simulink model "uz_ParameterID_6ph"  (R2021b)
settings: Solver=FixedStepDiscrete  StartTime=0.0  StopTime=160  FixedStep=0.000005  RelTol=1e-3  EnableMultiTasking=on
model workspace (MATLAB code in the model file):
  | cmdLim = Simulink.Parameter;
  | cmdLim.Value = 15;
  | cmdLim.Description = 'Limit for controlling the maximum surface command angle.';
  | cmdLim.Min = 0;
  | cmdLim.Max = 90;
  | cmdLim.DocUnits = 'deg';
  | 
  | dispGain = Simulink.Parameter;
  | dispGain.Value = 0.75;
  | dispGain.Description = 'Gain applied to the displacement error.';
  | dispGain.Min = 0;
  | dispGain.Max = [];
  | dispGain.DocUnits = 'deg/sec/deg';
  | 
  | dispLim = Simulink.Parameter;
  | dispLim.Value = 30;
  | dispLim.Description = 'Limit for controlling the maximum commanded angle.';
  | dispLim.Min = 0;
  | dispLim.Max = 180;
  | dispLim.DocUnits = 'deg';
  | 
  | intGain = Simulink.Parameter;
  | intGain.Value = 0.5;
  | intGain.Description = 'Gain applied to the integral error.';
  | intGain.Min = 0;
  | intGain.Max = [];
  | intGain.DocUnits = 'deg/sec/deg/sec';
  | 
  | intLim = Simulink.Parameter;
  | intLim.Value = 5;
  | intLim.Description = 'Limit for controlling the maximum commanded angle.';
  | intLim.Min = 0;
  | intLim.Max = 90;
  | intLim.DocUnits = 'deg';
  | 
  | rateGain = Simulink.Parameter;
  | rateGain.Value = 2;
  | rateGain.Description = 'Gain applied to the rate error.';
  | rateGain.Min = 0;
  | rateGain.Max = [];
  | rateGain.DocUnits = 'deg/deg/sec';
  | 
  | rateLim = Simulink.Parameter;
  | rateLim.Value = 6;
  | rateLim.Description = 'Limit for controlling the maximum commanded angle.';
  | rateLim.Min = 0;
  | rateLim.Max = 180;
  | rateLim.DocUnits = 'deg/sec';
  | 
  | hdgGain = Simulink.Parameter;
  | hdgGain.Value = 0.015;
values from neighbouring files (symbols this model uses):
  d_f_states = 20000    [Parameter_Init_Buehler_201.m]
  d_I_n = 8    [Parameter_Init_Buehler_201.m]
  d_Ki_id = 162.47    [Parameter_Init_Buehler_201.m]
  d_Ki_iq = 162.47    [Parameter_Init_Buehler_201.m]
  d_Ki_n = 1.982    [Parameter_Init_Buehler_201.m]
  d_Kp_id = 0.369    [Parameter_Init_Buehler_201.m]
  d_Kp_iq = 0.369    [Parameter_Init_Buehler_201.m]
  d_Kp_n = 0.198    [Parameter_Init_Buehler_201.m]
  d_L_d = 0.00031    [Parameter_Init_Buehler_201.m]
  d_L_q = 0.00033    [Parameter_Init_Buehler_201.m]
  d_n_n = 3200    [Parameter_Init_Buehler_201.m]
  d_p = 4    [Parameter_Init_Buehler_201.m]
  d_psi_pm = 0.0075    [Parameter_Init_Buehler_201.m]
  d_R_ph = d_R_ph_ph/2    (= 0.089)    [Parameter_Init_Buehler_201.m]
undefined symbols (not defined in the file or in its folder): i_dq_ref, n_ref
(part 1 of 2)
settings Model: RequirementInfo={} %GIDa_fe9045fd_0412_4b6e_8206_617cc20e6fde  FPTRunName=Active  Creator=ts  LastModifiedBy=valen
settings SolverCC: AlgebraicLoopSolver=TrustRegion  PositivePriorityOrder=on  AutoInsertRateTranBlk=on
settings DataIOCC: SaveOutput=off  SignalLogging=off  DSMLogging=off  SaveTime=off
settings OptimizationCC: DefaultParameterBehavior=Inlined  UseDivisionForNetSlopeComputation=on  GainParamInheritBuiltInType=on  UseFloatMulNetSlope=on  DefaultUnderspecifiedDataType=single  UseSpecifiedMinMax=on  InlineInvariantSignals=on  PassReuseOutputArgsAs=Individual arguments  ZeroExternalMemoryAtStartup=off  ZeroInternalMemoryAtStartup=off  NoFixptDivByZeroProtection=on  EfficientFloat2IntCast=on  LifeSpan=1  MaxStackSize=64  OptimizeBlockOrder=speed  DifferentSizesBufferReuse=on  EfficientTunableParamExpr=on
settings DebuggingCC: BusObjectLabelMismatch=error  AllowSymbolicDim=off  SFUnexpectedBacktrackingDiag=warning  SFNoUnconditionalDefaultTransitionDiag=warning  SFExecutionAtInitializationDiag=none  SFMachineParentedDataDiag=warning  ArithmeticOperatorsInVariantConditions=warning
settings HardwareCC: ProdBitPerPointer=32  ProdBitPerSizeT=32  ProdBitPerPtrDiffT=32  ProdLargestAtomicInteger=Long  ProdLargestAtomicFloat=Double  ProdWordSize=32  ProdLongLongMode=on  ProdHWDeviceType=ARM Compatible->ARM Cortex-R  HardwareBoardFeatureSet=SoCBlockset
settings SFSimCC: SimGenImportedTypeDefs=on  MATLABDynamicMemAlloc=off
settings RTWCC: Description=Embedded Coder  SystemTargetFile=ert.tlc  GenCodeOnly=on  TemplateMakefile=ert_default_tmf  GenerateReport=on  BuildConfiguration=Faster Runs  IncludeHyperlinkInReport=on  LaunchReport=on  GenerateTraceInfo=on  GenerateTraceReport=on  GenerateTraceReportSl=on  GenerateTraceReportSf=on  GenerateTraceReportEml=on  GenerateCodeMetricsReport=on  CheckMdlBeforeBuild=Warning
settings CodeAppCC: ForceParamTrailComments=on  IgnoreCustomStorageClasses=off  OperatorAnnotations=on  SimulinkDataObjDesc=on  SFDataObjDesc=on  MATLABFcnDesc=on  CustomSymbolStrGlobalVar=rt$M$R$N  CustomSymbolStrType=$N$M$R_t  CustomSymbolStrFcn=$N$M$F  CustomSymbolStrMacro=$N$M  InsertBlockDesc=on  StateflowObjectComments=on  MATLABSourceComments=on  EnableCustomComments=on  ReqsInCode=on
settings ERTTargetCC: TargetLangStandard=C99 (ISO)  CodeReplacementLibrary=GNU C99 extensions  MultiwordLength=2048  IncludeMdlTerminateFcn=off  CombineSignalStateStructs=on  SuppressErrorStatus=on  IncludeFileDelimiter=UseQuote  SupportAbsoluteTime=off  CodeInterfacePackaging=Reusable function  RemoveResetFunc=off  InlinedParameterPlacement=NonHierarchical  MultiInstanceErrorCode=Warning  RootIOFormat=Part of model data structure  ERTCustomFileTemplate=example_file_process.tlc  GlobalDataDefinition=InSourceFile  GlobalDataReference=InSourceFile  ERTFilePackagingFormat=CompactWithDataFile
settings ConfigComp: CovScope=ReferencedModels  CovSaveName=covdata_rollAP  CovMetricSettings=dcmtrwe  CovHTMLOptions=-sRT=1 -aTS=1 -bRG=1 -bTC=1 -hTR=1 -nFC=0 -scm=1 -bcm=1 -xEv=0  CovSaveCumulativeToWorkspaceVar=on  CovSaveSingleToWorkspaceVar=on  CovCumulativeVarName=covCumulativeData_rollAP  CovReportOnPause=off  CovExternalEMLEnable=off  CovSFcnEnable=off

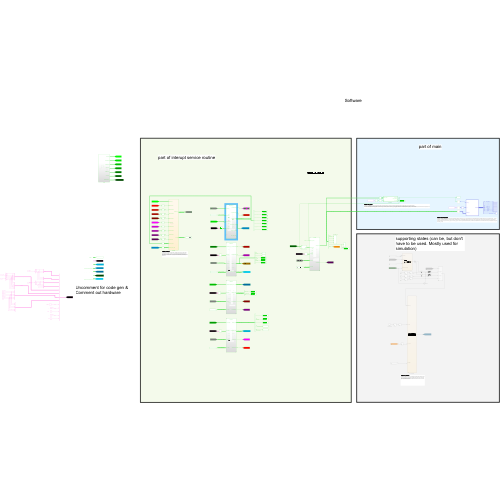
[thumbnail: Simulink's stored preview of the top-level diagram]
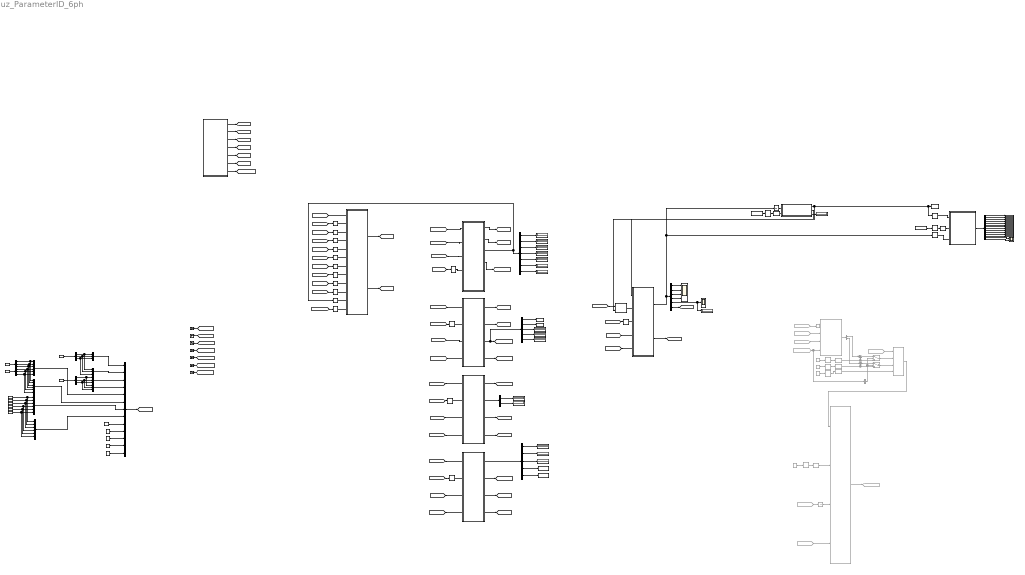
== system uz_ParameterID_6ph ==
  note: Description of Interpoaltion_Mesh_Grid:
      |
      | This function is calculating the regular flux maps out of the irregular scatter data array stored in psi_array_in. The outputs rangeX are containg the flux maps axis information, whereby the range is related to 3 times "i_rat" input.
      | Furthermore, the temperature dependency of the permanent flux is calculated if there are enough measuring values stored in the "delta_psi" array. The temperature constant as well as the estimated error of permanent flux,
      | at reference temperature, are given out on "psi_temp_const" and "psi_temp_error" outputs. Using this temperature dependency, the flux maps are updated with the permanent flux offset caused by the temperature which is given
      | in on "Wtemp_in" input.
  note: Stateflow for OnlineID
  note: part of main
  note: part of interupt service routine
  note: Software
  note: Description of clean_psi_array:
      |
      | This function is cleaning the array storing the measurement values, which always consits of a d-q-current combination a winding temperature and a speed value such as a d-q-flux combination
      | The function is searching for measuring pairs which are closer than "eta_c" to their neighbours. In this case it is averaging this similar pairs to avoid measuring values containing the same information.
      | This is essential for calculating a wide ranging flux map out of this array. Furthermore, there is an output "n_flux_points" giving back the amount of independent measuring pairs. This is the number (x/100) i show in the JavaGUI on the rigth top corner.
  note: Uncomment for code gen & Comment out hardware
  note: Description of ControlState:
      |
      | This state includes controls all the other states. It decides, based on user input, which state is executed and in which order. This is done via ControlFlags and finished/entered Flags of the individual states. If multiple ID's are requested, this state will automatically start the next one after the previous one has finished. This is an integral part of the ParameterID and must always be implemented.
  note: Description FOC_ControlState:
      |
      | This Stateflow is entered, after every other ID-state is finished (except OnlineID). It's just a simple state for current & speed control, depending on what the user chose in the config. This is only used to control the FOC with inputs after the ID-states are done. This state is solely used for simulation purposes.
  note: supporting states (can be, but don't have to be used. Mostly used for simulation)
  0 = current control 1 = speed control : Constant  Commented=on  Value=0
  AutoRefCurrents : Stateflow chart  Commented=on  TreatAsAtomicUnit=on
      settings: PortSchema="{\"entries\":[{\"content\":{\"sides\":[{\"content\":{\"connectorIds\":[\"In1\",\"In2\",\"In4\",\"In3\"]},\"type\":\"ConnectorPlacement.EquallySpacedRectSide\",\"uuid\":\"72ec0a24-315d-4dd0-9768-288ce3b452e0\"},{\"content\":{\"connectorIds\":[\"Out1\"],\"side\":\"RIGHT\"},\"type\":\"ConnectorPlacement.EquallySpacedRectSide\",\"uuid\":\"ab2b6233-d9cb-4afd-91e6-1fd664e04fd4\"},{\"content\":{\"connectorIds\":[],\"side\":\"TOP\"},\"type\":\"ConnectorPlacement.EquallySpacedRectSide\",\"uuid\":\"64b2df27-0928-499d-b44c-d4351b3511f9\"}]},\"type\":\"ConnectorPlacement.EquallySpacedConnector\",\"uuid\":\"4bb55e1f-14f7-4ef2-bb52-ee940a9b3e5d\"}],\"packageUris\":[\"http://schema.mathworks.com/mf0/Connector/R2020b\"],\"version\":\"1.0\"}"
  Bus Assignment : BusAssignment  Commented=on  AssignedSignals=i_dq_ref.d,i_dq_ref.q,n_ref
  Bus Assignment1 : BusAssignment  AssignedSignals=array_cleaned
  Bus Creator : BusCreator  Inputs=13  OutDataTypeStr=Bus: uz_ParaID_ActualValues_t
  Bus Creator1 : BusCreator  Inputs=3  OutDataTypeStr=Bus: uz_3ph_abc_t
  Bus Creator10 : BusCreator  Inputs=6  OutDataTypeStr=Bus: uz_6ph_abc_t
  Bus Creator11 : BusCreator  Inputs=6  OutDataTypeStr=Bus: uz_6ph_abc_t
  Bus Creator2 : BusCreator  Inputs=3  OutDataTypeStr=Bus: uz_3ph_abc_t
  Bus Creator3 : BusCreator  Inputs=6  OutDataTypeStr=Bus: uz_6ph_dq_t
  Bus Creator4 : BusCreator  Inputs=6  OutDataTypeStr=Bus: uz_6ph_dq_t
  Bus Creator5 : BusCreator  Inputs=3  OutDataTypeStr=Bus: uz_3ph_dq_t
  Bus Creator6 : BusCreator  Inputs=3  OutDataTypeStr=Bus: uz_3ph_dq_t
  Bus Selector : BusSelector  OutputSignals=BrkTorque,CoulTorque,ViscoTorque,measArrayTorque,measArraySpeed
  Bus Selector2 : BusSelector  OutputSignals=thetaOffset,PMSM_parameters.R_ph_Ohm,PMSM_parameters.Ld_Henry,PMSM_parameters.Lq_Henry,PMSM_parameters.Psi_PM_Vs,PMSM_parameters.J_kg_m_squared,PMSM_parameters.polePairs
  Bus Selector3 : BusSelector  OutputSignals=range_psid_X,range_psiq_X,range_id_X,range_iq_X,range_psid_Y,range_psiq_Y,range_id_Y,range_iq_Y,psiq_grid,psid_grid,id_grid,iq_grid,psi_temp_const,psi_temp_error
  Bus Selector4 : BusSelector  Commented=on  OutputSignals=i_dq_ref.d,i_dq_ref.q
  Bus Selector5 : BusSelector  OutputSignals=R_s,WindingTemp
  Bus Selector6 : BusSelector  OutputSignals=c_est_out,d_est_out,LoadInertia,TrainInertia,rotorInertia
  Bus Selector7 : BusSelector  Commented=on  OutputSignals=enableCRS
  Bus Selector8 : BusSelector  OutputSignals=Rph_out,Ld_out,Lq_out,psi_pm_out,activeState,id_out
  CleanPsiArray : MATLAB Function
  Const27 : Constant  Value=0.01*d_I_n
  Const53 : Constant  Value=d_I_n
  Const7 : Constant  Commented=on  Value=0.6
  Const8 : Constant  Commented=on  Value=0
  Const9 : Constant  Commented=on  Value=1000
  Constant{,2..5,7} (6 alike) : Constant  Value=0  OutDataTypeStr=single
  Constant{1,6,16..17} (4 alike) : Constant  Value=[0;0;0]  OutDataTypeStr=single
  ControlState : Stateflow chart  TreatAsAtomicUnit=on
      settings: PortSchema="{\"entries\":[{\"content\":{\"sides\":[{\"content\":{\"connectorIds\":[\"In11\",\"In1\",\"In2\",\"In3\",\"In4\",\"In5\",\"In8\",\"In7\",\"In6\",\"In12\",\"In9\",\"In10\"]},\"type\":\"ConnectorPlacement.EquallySpacedRectSide\",\"uuid\":\"3338e9a8-28b4-45bb-be16-581ebbf0e7d5\"},{\"content\":{\"connectorIds\":[\"Out1\",\"Out2\"],\"side\":\"RIGHT\"},\"type\":\"ConnectorPlacement.EquallySpacedRectSide\",\"uuid\":\"68ffdf0a-d88e-422d-a36e-256c991e1a1a\"},{\"content\":{\"connectorIds\":[],\"side\":\"TOP\"},\"type\":\"ConnectorPlacement.EquallySpacedRectSide\",\"uuid\":\"571bf6fb-233c-470d-b735-d23e4cf83e69\"}]},\"type\":\"ConnectorPlacement.EquallySpacedConnector\",\"uuid\":\"829c5db0-50d3-4caf-9d4e-ee907b3905d4\"}],\"packageUris\":[\"http://schema.mathworks.com/mf0/Connector/R2020b\"],\"version\":\"1.0\"}"
  Data Type Conversion107 : DataTypeConversion  Commented=on  OutDataTypeStr=boolean
  Data Type Conversion12 : DataTypeConversion  Commented=on  OutDataTypeStr=single
  Data Type Conversion13 : DataTypeConversion  Commented=on  OutDataTypeStr=single
  Data Type Conversion15 : DataTypeConversion  Commented=on  OutDataTypeStr=single
  Data Type Conversion60 : DataTypeConversion  OutDataTypeStr=single
  Data Type Conversion86 : DataTypeConversion  OutDataTypeStr=single
  Delay{,1..9,14} (11 alike) : Delay  DelayLength=1  InitialCondition=0
  Demux{1..4} (4 alike) : Demux  Outputs=3
  Display{1..3,5..11} (10 alike) : Display
  ElectricalID6ph : Subsystem  ReferencedSubsystem=ElectricalID_6ph
  FOC_ControlState : Stateflow chart  Commented=on  TreatAsAtomicUnit=on
      settings: PortSchema="{\"entries\":[{\"content\":{\"sides\":[{\"content\":{\"connectorIds\":[\"In2\",\"In4\",\"In1\",\"In3\"]},\"type\":\"ConnectorPlacement.EquallySpacedRectSide\",\"uuid\":\"51616e24-a97c-4867-a832-fbf8995ba5af\"},{\"content\":{\"connectorIds\":[\"Out1\"],\"side\":\"RIGHT\"},\"type\":\"ConnectorPlacement.EquallySpacedRectSide\",\"uuid\":\"f89ef2d6-1fe7-4143-9573-492fc01180c7\"},{\"content\":{\"connectorIds\":[],\"side\":\"TOP\"},\"type\":\"ConnectorPlacement.EquallySpacedRectSide\",\"uuid\":\"2a1663ee-9e4b-4188-8f87-b811d0bf4173\"}]},\"type\":\"ConnectorPlacement.EquallySpacedConnector\",\"uuid\":\"7415555a-a8a9-4dd7-91ae-86382220971a\"}],\"packageUris\":[\"http://schema.mathworks.com/mf0/Connector/R2020b\"],\"version\":\"1.0\"}"
  From11 : From  Commented=on  GotoTag=OnlineID_id_out
  From39 : From  Commented=on  GotoTag=ActualValues
  From40 : From  Commented=on  GotoTag=GlobalConfig
  From5 : From  Commented=on  GotoTag=ControlFlags
  From50 : From  Commented=on  GotoTag=GlobalConfig
  From51 : From  Commented=on  GotoTag=AutoRefCurrentsConfig
  From52 : From  Commented=on  GotoTag=ControlFlags
  Goto8 : Goto  Commented=on  GotoTag=FOCControl_output
  InterpMeshGrid : MATLAB Function  TreatAsAtomicUnit=on
  OnlineActiveState : Scope
  RT : RateTransition  Commented=on  OutPortSampleTime=0.0001
  Rate Transition : RateTransition  OutPortSampleTime=0.1
  Rate Transition{1,13..14,147} (4 alike) : RateTransition  Commented=on  OutPortSampleTime=1/d_f_states
  Rate Transition{2..6,78} (6 alike) : RateTransition  OutPortSampleTime=1/d_f_states
  Rate Transition85 : RateTransition  OutPortSampleTime=0.1
  Rate Transition90 : RateTransition  OutPortSampleTime=0.1
  Rs,Ld,Lq,Psi_pm : Scope  NumInputPorts=4
  Scope2 : Scope  NumInputPorts=2
  Subsystem Reference : Subsystem  ReferencedSubsystem=FrictionID
  Subsystem Reference1 : Subsystem  ReferencedSubsystem=FluxMapID
  Subsystem Reference3 : Subsystem  ReferencedSubsystem=TwoMassID
  Subsystem Reference4 : Subsystem  ReferencedSubsystem=OnlineID
  Sum : Sum  Commented=on  Inputs=|++
  Sum1 : Sum  Commented=on  Inputs=|++
  Switch2 : Switch  Commented=on  Criteria=u2 > Threshold
  Switch3 : Switch  Commented=on  Criteria=u2 > Threshold
  Terminator{,1..6} (7 alike) : Terminator
  To Workspace1 : ToWorkspace  VariableName=measArrayTorque  SampleTime=-1
      settings: MaxDataPoints=1
  To Workspace15 : ToWorkspace  VariableName=psi_array  SampleTime=-1
      settings: MaxDataPoints=1
  To Workspace16 : ToWorkspace  VariableName=rangepdX  SampleTime=-1
      settings: MaxDataPoints=1
  To Workspace17 : ToWorkspace  VariableName=rangepqX  SampleTime=-1
      settings: MaxDataPoints=1
  To Workspace18 : ToWorkspace  VariableName=rangeidX  SampleTime=-1
      settings: MaxDataPoints=1
  To Workspace19 : ToWorkspace  VariableName=rangeiqX  SampleTime=-1
      settings: MaxDataPoints=1
  To Workspace2 : ToWorkspace  VariableName=measArraySpeed  SampleTime=-1
      settings: MaxDataPoints=1
  To Workspace20 : ToWorkspace  VariableName=rangepdY  SampleTime=-1
      settings: MaxDataPoints=1
  To Workspace21 : ToWorkspace  VariableName=rangepqY  SampleTime=-1
      settings: MaxDataPoints=1
  To Workspace22 : ToWorkspace  VariableName=rangeidY  SampleTime=-1
      settings: MaxDataPoints=1
  To Workspace23 : ToWorkspace  VariableName=rangeiqY  SampleTime=-1
      settings: MaxDataPoints=1
  To Workspace24 : ToWorkspace  VariableName=psiq_grid  SampleTime=-1
      settings: MaxDataPoints=1
  To Workspace25 : ToWorkspace  VariableName=psid_grid  SampleTime=-1
      settings: MaxDataPoints=1
  To Workspace26 : ToWorkspace  VariableName=id_grid  SampleTime=-1
      settings: MaxDataPoints=1
  To Workspace27 : ToWorkspace  VariableName=iq_grid  SampleTime=-1
      settings: MaxDataPoints=1
  To Workspace31 : ToWorkspace  VariableName=c_est_out  SampleTime=-1
      settings: MaxDataPoints=1
  To Workspace32 : ToWorkspace  VariableName=d_est_out  SampleTime=-1
      settings: MaxDataPoints=1
  Unit Delay : UnitDelay  Commented=on  SampleTime=-1  HasFrameUpgradeWarning=on
  Unit Delay3 : UnitDelay  SampleTime=-1  HasFrameUpgradeWarning=on
  V_DC : Constant  Value=0  OutDataTypeStr=single
  config : Subsystem
  d-axis inductance Ld [H] : Display
  omega_el : Constant  Value=0  OutDataTypeStr=single
  omega_m : Constant  Value=0  OutDataTypeStr=single
  p : Display
  phase resistance [Ohm] : Display
  psiPM [Vs] : Display
  q-axis inductance Lq [H] : Display
  rotorInertia  [kg*m²] : Display
  thetaOffset [rad] : Display
  theta_el : Constant  Value=0  OutDataTypeStr=single
  theta_m : Constant  Value=0  OutDataTypeStr=single
  wires:
  Bus Selector/3 -> Display10/1  "<ViscoTorque>"
  Sum/1 -> Switch3/1
  Const8/1 -> Rate Transition13/1
  config/5(TwoMassIDConfig) -> [TwoMassIDConfig]
  Bus Selector2/4 -> q-axis inductance Lq [H]/1  "<Lq_Henry>"
  From40/1 -> AutoRefCurrents/2(GlobalConfig)
  [finishedFrictionID] -> Delay/1
  Delay/1 -> ControlState/1(finishedFrictionID)
  Bus Selector2/5 -> psiPM [Vs]/1  "<Psi_PM_Vs>"
  Bus Selector8/1 -> Rs,Ld,Lq,Psi_pm/1  "<Rph_out>"
  Bus Selector6/5 -> Display6/1  "<rotorInertia>"
  Sum1/1 -> Switch2/1
  Const9/1 -> Rate Transition1/1
  Rate Transition14/1 -> Data Type Conversion13/1
  config/1(GlobalConfig) -> [GlobalConfig_in]
  Delay14/1 -> ControlState/9(ElectricalID_output)
  Delay2/1 -> ControlState/6(enteredFluxMapID)
  Delay5/1 -> ControlState/8(enteredElectricalID)
  Delay6/1 -> ControlState/7(enteredTwoMassID)
  [enteredElectricalID] -> Delay5/1
  Rate Transition85/1 -> Data Type Conversion86/1
  [enteredFrictionID] -> Delay1/1
  Data Type Conversion13/1 -> Sum1/2, Switch2/3  "i_q_ref"
  Rate Transition90/1 -> InterpMeshGrid/3(OnlineID_input)
  [finishedFluxMapID] -> Delay4/1
  [finishedTwoMassID] -> Delay3/1
  From39/1 -> RT/1
  config/2(ElectricalIDConfig) -> [ElectricalIDConfig]
  config/4(FrictionIDConfig) -> [FrictionIDConfig]
  Const53/1 -> Rate Transition85/1
  Const27/1 -> Rate Transition78/1
  Data Type Conversion60/1 -> CleanPsiArray/2(eta_c)
  Bus Selector2/6 -> rotorInertia  [kg*m²]/1  "<J_kg_m_squared>"
  Bus Selector/1 -> Display11/1  "<BrkTorque>"
  Delay1/1 -> ControlState/5(enteredFrictionID)
  Bus Selector2/7 -> p/1  "<polePairs>"
  [ElectricalID_FOC_output] -> Delay8/1
  Rate Transition13/1 -> Data Type Conversion12/1
  Unit Delay/1 -> FOC_ControlState/1(i_d_Online_ref)
  Rate Transition/1 -> InterpMeshGrid/1(psi_array_in)
  Delay7/1 -> ControlState/2(finishedElectricalID)
  Bus Selector2/2 -> phase resistance [Ohm]/1  "<R_ph_Ohm>"
  Bus Selector2/3 -> d-axis inductance Ld [H]/1  "<Ld_Henry>"
  [ActualValues] -> Rate Transition6/1
  Delay8/1 -> ControlState/10(ElectricalID_FOC_output)
  Bus Selector6/3 -> Display3/1  "<LoadInertia>"
  ControlState/1(GlobalConfig_out) -> [GlobalConfig]
  [ActualValues] -> Rate Transition2/1
  config/6(OnlineIDConfig) -> [OnlineIDConfig]
  [ActualValues] -> Rate Transition3/1
  CleanPsiArray/2(array_cleaned_flag) -> Bus Assignment1/2
  Bus Selector5/1 -> Display1/1  "<R_s>"
  [GlobalConfig_in] -> ControlState/11(GlobalConfig_in)
  From5/1 -> FOC_ControlState/3(ControlFlags)
  Const7/1 -> Rate Transition14/1
  Bus Selector6/4 -> Display5/1  "<TrainInertia>"
  Data Type Conversion86/1 -> InterpMeshGrid/2(i_rat)
  Bus Selector8/4 -> Rs,Ld,Lq,Psi_pm/4  "<psi_pm_out>"
  Bus Selector8/2 -> Rs,Ld,Lq,Psi_pm/2  "<Ld_out>"
  Unit Delay3/1 -> CleanPsiArray/1(OnlineID_output)
  [OnlineIDConfig] -> Bus Assignment1/1
  Rate Transition78/1 -> Data Type Conversion60/1
  Rate Transition1/1 -> Data Type Conversion15/1
  Bus Selector8/5 -> Display8/1, OnlineActiveState/1  "<activeState>"
  Delay3/1 -> ControlState/3(finishedTwoMassID)
  CleanPsiArray/1(psi_array_out) -> Subsystem Reference4/1, Rate Transition/1, To Workspace15/1  "cleaned_psi_array"
  Bus Selector2/1 -> thetaOffset [rad]/1  "<thetaOffset>"
  config/3(FluxMapIDConfig) -> [FluxMapIDConfig]
  CleanPsiArray/3(n_flux_points) -> Display7/1
  Bus Selector/2 -> Display9/1  "<CoulTorque>"
  ControlState/2(ControlFlags) -> [ControlFlags]
  [ActualValues] -> Rate Transition4/1
  Bus Selector6/1 -> To Workspace31/1  "<c_est_out>"
  Bus Selector6/2 -> To Workspace32/1  "<d_est_out>"
  FOC_ControlState/1(FOCControl_output) -> Goto8/1
  Delay4/1 -> ControlState/4(finishedFluxMapID)
  [finishedElectricalID] -> Delay7/1
  Bus Assignment/1 -> FOC_ControlState/2(GlobalConfig)
  [ActualValues] -> Rate Transition5/1
  Bus Selector8/3 -> Rs,Ld,Lq,Psi_pm/3  "<Lq_out>"
  Data Type Conversion12/1 -> Switch3/3, Sum/2  "i_d_ref"
  [enteredFluxMapID] -> Delay2/1
  [enteredTwoMassID] -> Delay6/1
  Bus Selector5/2 -> Display2/1  "<WindingTemp>"
  [ActualValues] -> Terminator/1
  [TwoMassID_FOC_output] -> Terminator6/1
  [FrictionID_FOC_output] -> Terminator2/1
  [ElectricalID_FOC_output] -> Terminator3/1
  [FluxMapID_FOC_output] -> Terminator4/1
  [ControlFlags] -> Terminator1/1
  omega_el/1 -> Bus Creator/10  "omega_el"
  Bus Creator/1 -> [ActualValues]
  omega_m/1 -> Bus Creator/9  "omega_m"
  theta_m/1 -> Bus Creator/11  "theta_m"
  V_DC/1 -> Bus Creator/13  "V_DC"
  theta_el/1 -> Bus Creator/12  "theta_el"
  From50/1 -> Bus Assignment/1
  Switch2/1 -> Bus Assignment/3
  Switch3/1 -> Bus Assignment/2
  Data Type Conversion15/1 -> Bus Assignment/4  "n_ref"
  RT/1 -> AutoRefCurrents/1(ActualValues)
  Bus Selector8/6 -> [OnlineID_id_out]  "<id_out>"
  From11/1 -> Unit Delay/1
  Rate Transition147/1 -> Data Type Conversion107/1
  Data Type Conversion107/1 -> FOC_ControlState/4(controlType)  "controlType"
  0 = current control 1 = speed control/1 -> Rate Transition147/1
  Bus Selector3/1 -> To Workspace16/1  "<range_psid_X>"
  Bus Selector3/2 -> To Workspace17/1  "<range_psiq_X>"
  InterpMeshGrid/1(FluxMapData) -> Bus Selector3/1
  Bus Selector3/14 -> Scope2/2  "<psi_temp_error>"
  Bus Selector3/13 -> Scope2/1  "<psi_temp_const>"
  Bus Selector3/3 -> To Workspace18/1  "<range_id_X>"
  Bus Selector3/4 -> To Workspace19/1  "<range_iq_X>"
  Bus Selector3/5 -> To Workspace20/1  "<range_psid_Y>"
  Bus Selector3/6 -> To Workspace21/1  "<range_psiq_Y>"
  Bus Selector3/7 -> To Workspace22/1  "<range_id_Y>"
  Bus Selector3/8 -> To Workspace23/1  "<range_iq_Y>"
  Bus Selector3/9 -> To Workspace24/1  "<psiq_grid>"
  Bus Selector3/10 -> To Workspace25/1  "<psid_grid>"
  Bus Selector3/11 -> To Workspace26/1  "<id_grid>"
  Bus Selector3/12 -> To Workspace27/1  "<iq_grid>"
  config/7(AutoRefCurrentsconfig) -> [AutoRefCurrentsConfig]
  From51/1 -> Bus Selector7/1, AutoRefCurrents/3(AutoRefCurrentsConfig)
  AutoRefCurrents/1(AutoRefCurrents_output) -> Bus Selector4/1
  Bus Selector4/1 -> Sum/1  "<d>"
  Bus Selector4/2 -> Sum1/1  "<q>"
  Bus Selector7/1 -> Switch2/2, Switch3/2  "<enableCRS>"
  From52/1 -> AutoRefCurrents/4(ControlFlags)
  Delay9/1 -> ControlState/12(enteredOnlineID)
  [enteredOnlineID] -> Delay9/1
  Bus Selector/4 -> To Workspace1/1  "<measArrayTorque>"
  Bus Selector/5 -> To Workspace2/1  "<measArraySpeed>"
  [FrictionIDConfig] -> Subsystem Reference/1
  [GlobalConfig] -> Subsystem Reference/3
  [ControlFlags] -> Subsystem Reference/4
  Subsystem Reference/1 -> Bus Selector/1
  Subsystem Reference/2 -> [FrictionID_FOC_output]
  Subsystem Reference/3 -> [enteredFrictionID]
  Subsystem Reference/4 -> [finishedFrictionID]
  [FluxMapIDConfig] -> Subsystem Reference1/1
  [GlobalConfig] -> Subsystem Reference1/3
  [ControlFlags] -> Subsystem Reference1/4
  Subsystem Reference1/1 -> [FluxMapID_FOC_output]
  Subsystem Reference1/2 -> Bus Selector5/1
  Subsystem Reference1/3 -> [finishedFluxMapID]
  Subsystem Reference1/4 -> [enteredFluxMapID]
  ElectricalID6ph/3 -> Bus Selector2/1, Delay14/1
  [GlobalConfig] -> ElectricalID6ph/1
  [ControlFlags] -> ElectricalID6ph/2
  [ElectricalIDConfig] -> ElectricalID6ph/3
  Rate Transition6/1 -> ElectricalID6ph/4
  ElectricalID6ph/1 -> [enteredElectricalID]
  ElectricalID6ph/2 -> [finishedElectricalID]
  ElectricalID6ph/4 -> [ElectricalID_FOC_output]
  Subsystem Reference3/3 -> Bus Selector6/1, [TwoMassID_output]
  [TwoMassIDConfig] -> Subsystem Reference3/1
  [GlobalConfig] -> Subsystem Reference3/3
  [ControlFlags] -> Subsystem Reference3/4
  Subsystem Reference3/1 -> [finishedTwoMassID]
  Subsystem Reference3/2 -> [enteredTwoMassID]
  Subsystem Reference3/4 -> [TwoMassID_FOC_output]
  Subsystem Reference4/1 -> Unit Delay3/1, Rate Transition90/1, Bus Selector8/1
  Bus Assignment1/1 -> Subsystem Reference4/2
  Rate Transition3/1 -> Subsystem Reference4/3
  [GlobalConfig] -> Subsystem Reference4/4
  [ControlFlags] -> Subsystem Reference4/5
  Subsystem Reference4/2 -> [enteredOnlineID]
  Rate Transition2/1 -> Subsystem Reference3/2
  Rate Transition4/1 -> Subsystem Reference1/2
  Rate Transition5/1 -> Subsystem Reference/2
  Demux1/3 -> Bus Creator11/3, Bus Creator10/3  "c1"
  Demux1/2 -> Bus Creator11/2, Bus Creator10/2  "b1"
  Constant17/1 -> Demux2/1
  Constant16/1 -> Demux1/1
  Demux2/1 -> Bus Creator11/4, Bus Creator10/4  "a2"
  Demux2/3 -> Bus Creator11/6, Bus Creator10/6  "c2"
  Demux1/1 -> Bus Creator11/1, Bus Creator10/1  "a1"
  Demux2/2 -> Bus Creator11/5, Bus Creator10/5  "b2"
  Bus Creator11/1 -> Bus Creator/6  "i_abc_6ph"
  Bus Creator10/1 -> Bus Creator/5  "v_abc_6ph"
  Constant2/1 -> Bus Creator3/2, Bus Creator4/2  "q"
  Constant3/1 -> Bus Creator3/3, Bus Creator4/3  "x"
  Constant/1 -> Bus Creator3/1, Bus Creator4/1  "d"
  Bus Creator4/1 -> Bus Creator/7  "i_dq_6ph"
  Constant4/1 -> Bus Creator3/4, Bus Creator4/4  "y"
  Bus Creator3/1 -> Bus Creator/8  "v_dq_6ph"
  Constant5/1 -> Bus Creator3/5, Bus Creator4/5  "z1"
  Constant7/1 -> Bus Creator3/6, Bus Creator4/6  "z2"
  Demux3/3 -> Bus Creator2/3, Bus Creator1/3  "c"
  Demux3/1 -> Bus Creator2/1, Bus Creator1/1  "a"
  Demux3/2 -> Bus Creator2/2, Bus Creator1/2  "b"
  Constant1/1 -> Demux3/1
  Bus Creator1/1 -> Bus Creator/1  "V_abc"
  Bus Creator2/1 -> Bus Creator/2  "I_abc"
  Bus Creator5/1 -> Bus Creator/3  "i_dq"
  Constant6/1 -> Demux4/1
  Demux4/3 -> Bus Creator6/3, Bus Creator5/3  "zero"
  Demux4/1 -> Bus Creator6/1, Bus Creator5/1  "d"
  Demux4/2 -> Bus Creator6/2, Bus Creator5/2  "q"
  Bus Creator6/1 -> Bus Creator/4  "v_dq"
  [AutoRefCurrentsConfig] -> Terminator5/1

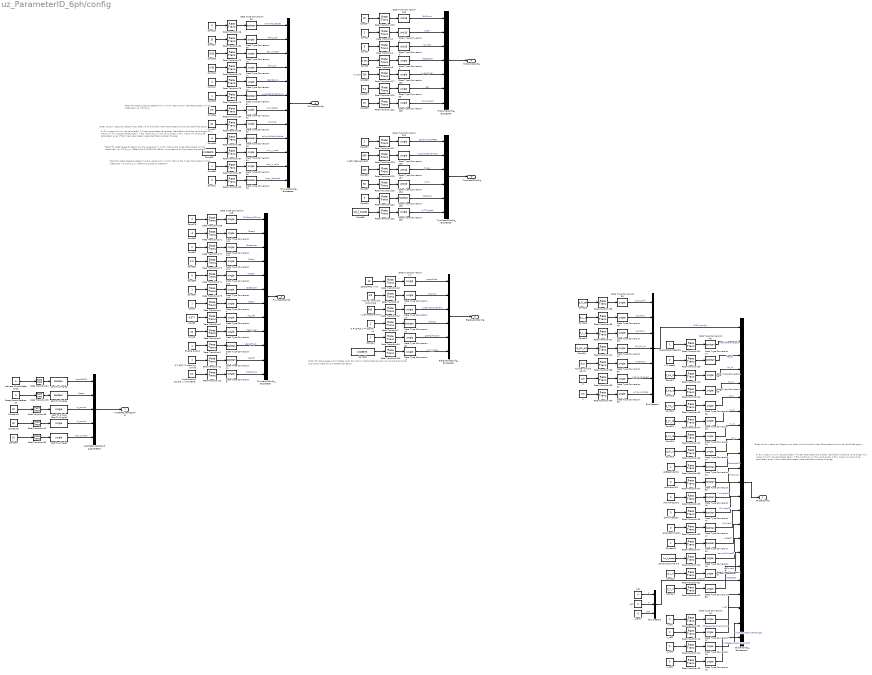
== system uz_ParameterID_6ph/config ==
  note: %1000
  note: Factor for rated speed,to determine the upper end in which interval the linear Parameters will
      | be measured. i.e. 0,5*d_n_n.
      | Default ist 0.625 for 2000rpm
  note: 0: Flux maps will only be calculated, if linear parameters have been identified inside the valid range.
      |     Flux maps will only be calculated again, if the machine is in the valid range.
      | 1:Flux maps will always be calculated, even if the linear parameters were identified outside of range.
  note: Enter value in seconds. Determines, after which time the linear Parameters have to be identified again.
  note: Factor for rated current,to determine in which interval the linear Parameters will
      | be measured. i.e. 0,5*d_I_n
  note: Factor for rated speed,to determine the lower end in which interval the linear Parameters will
      | be measured. i.e. 0,5*d_n_n.
      | Default ist 0.026875 for 86rpm (one rotation during measuring period)
  note: Factor for rated speed,which states when the rotor is rotating fast enough during the DutyCycle evaluation
      | Default ist 0.026875 for 86rpm
  note: 0: Flux maps will only be calculated, if linear parameters have been identified inside the valid range.
      |     Flux maps will only be calculated again, if the machine is in the valid range.
      | 1:Flux maps will always be calculated, even if the linear parameters were identified outside of range.
  note: Enter value in seconds. Determines, after which time the linear Parameters have to be identified again.
  "0 = Lq=Ld 1 = identify Lq " : Constant
  0 = off 1 = ident R_s online : Constant
  1 = reset1 : Constant  Value=0
  2 : Constant  Value=0.0
  3 : Constant  Value=0.0
  Activate ControlReference : Constant  Value=0  OutDataTypeStr=boolean
  Amplitude for SquareWave signal in d-current2 : Constant  Value=0.2
  AutoRefCurrentsConfig_Buscreator : BusCreator  Inputs=5  OutDataTypeStr=Bus: uz_ParaID_AutoRefCurrentsConfig_t
  Bus Creator1 : BusCreator  Inputs=7  OutDataTypeStr=Bus: uz_PMSM_t
  Bus Creator2 : BusCreator  Inputs=3  OutDataTypeStr=Bus: uz_3ph_dq_t
  Cast To Single : DataTypeConversion  OutDataTypeStr=single
  Cast To Single1 : DataTypeConversion  OutDataTypeStr=single
  Cast To Single2 : DataTypeConversion  OutDataTypeStr=single
  Cast To Single3 : DataTypeConversion  OutDataTypeStr=boolean
  Cast To Single4 : DataTypeConversion  OutDataTypeStr=boolean
  Const{1,47,78,81,91} (5 alike) : Constant  Value=2
  Const{10..11,58,83,94} (5 alike) : Constant  Value=0
  Const12 : Constant  Value=d_psi_pm
  Const13 : Constant  Value=d_I_n
  Const14 : Constant  Value=d_n_n
  Const16 : Constant  Value=d_L_d
  Const17 : Constant  Value=d_Kp_id
  Const18 : Constant  Value=d_Kp_iq
  Const19 : Constant  Value=d_Ki_iq
  Const2 : Constant  Value=5
  Const{4,20,28,60,84} (5 alike) : Constant
  Const21 : Constant  Value=d_Ki_id
  Const22 : Constant  Value=d_Kp_n
  Const23 : Constant  Value=d_Ki_n
  Const24 : Constant  Value=d_L_q
  Const25 : Constant  Value=d_R_ph
  Const3 : Constant  Value=0.001
  Const37 : Constant  Value=20
  Const43 : Constant  Value=0.05
  Const44 : Constant  Value=0.05
  Const5 : Constant  Value=0.077
  Const56 : Constant  Value=0.5
  Const57 : Constant  Value=20
  Const59 : Constant  Value=0.026875
  Const6 : Constant  Value=22
  Const62 : Constant  Value=0.026875
  Const64 : Constant  Value=0.2
  Const65 : Constant  Value=200
  Const67 : Constant  Value=20
  Const69 : Constant  Value=15
  Const80 : Constant  Value=-2
  Const82 : Constant  Value=0.0
  Const92 : Constant  Value=50
  Const93 : Constant  Value=400
  Const95 : Constant  Value=1/d_f_states
  Constant : Constant  Value=10
  Constant1 : Constant
  Constant3 : Constant  Value=20
  Constant4 : Constant  Value=20
  Data Type Conversion{1..2,103,136..137} (5 alike) : DataTypeConversion  OutDataTypeStr=uint16
  Data Type Conversion{8,10..11,23..24,26,40..41,43,47..48,54..55,61,93,138} (16 alike) : DataTypeConversion  OutDataTypeStr=boolean
  Data Type Conversion{3..7,9,12..15,17,25,33..39,42,45..46,49..53,56..58,76..77,80,91..92,94..95,97,99..100,105,118,120..124,134..135,139} (50 alike) : DataTypeConversion  OutDataTypeStr=single
  ElectricalIDConfig_Buscreater : BusCreator  Inputs=6  OutDataTypeStr=Bus: uz_ParaID_ElectricalIDConfig_t
  Enable output : Constant
  FluxMapIDConfig_Buscreater : BusCreator  Inputs=12  OutDataTypeStr=Bus: uz_ParaID_FluxMapIDConfig_t
  FrictionIDConfig_Buscreater : BusCreator  Inputs=7  OutDataTypeStr=Bus: uz_ParaID_FrictionIDConfig_t
  GlobalConfig_Buscreator1 : BusCreator  Inputs=23  OutDataTypeStr=Bus: uz_ParaID_GlobalConfig_t
  ISR sample time 0.2 : Constant  Value=1/d_f_states
  Number of pole pairs1 : Constant  Value=d_p
  OnlineIDConfig_Buscreater : BusCreator  Inputs=12  OutDataTypeStr=Bus: uz_ParaID_OnlineIDConfig_t
  Rate Transition{1..15,18,23..26,33..48,50..62,72..73,76,79,88,94..98,100,116..117,120,122,169,171..175,217..222} (76 alike) : RateTransition  OutPortSampleTime=1/d_f_states
  Reset ControlReference : Constant  Value=0  OutDataTypeStr=boolean
  TwoMassIDConfig_Buscreater : BusCreator  Inputs=6  OutDataTypeStr=Bus: uz_ParaID_TwoMassIDConfig_t
  doElectricalID1 : Constant
  doFluxMapID1 : Constant  Value=0
  doFrictionID1 : Constant  Value=0
  doTwoMassID1 : Constant  Value=0
  enableOnlineID1 : Constant  Value=0
  enableParameterID1 : Constant
  goertzlFreq in Hz : Constant  Value=40
  i_d1 : Constant  Value=0  OutDataTypeStr=single
  i_q1 : Constant  Value=0  OutDataTypeStr=single
  i_zero1 : Constant  Value=0  OutDataTypeStr=single
  manual input of a DutyCycle : Constant  Value=0.5
  n_ref measurement : Constant  Value=500
  n_ref measurement1 : Constant  Value=400
  n_ref{1..4} (4 alike) : Constant  Value=0
  GlobalConfig : Outport
  ElectricalIDConfig : Outport  Port=2
  FluxMapIDConfig : Outport  Port=3
  FrictionIDConfig : Outport  Port=4
  TwoMassIDConfig : Outport  Port=5
  OnlineIDConfig : Outport  Port=6
  AutoRefCurrentsconfig : Outport  Port=7
  wires:
  Data Type Conversion1/1 -> FrictionIDConfig_Buscreater/2  "N_Brk"
  Data Type Conversion99/1 -> FrictionIDConfig_Buscreater/6  "eta"
  Data Type Conversion2/1 -> FrictionIDConfig_Buscreater/3  "N_Visco"
  Data Type Conversion103/1 -> FrictionIDConfig_Buscreater/1  "BrkCount"
  Data Type Conversion105/1 -> FrictionIDConfig_Buscreater/7  "maxCurrent"
  Data Type Conversion100/1 -> FrictionIDConfig_Buscreater/5  "n_eva_max"
  Data Type Conversion3/1 -> FrictionIDConfig_Buscreater/4  "StepScale"
  FrictionIDConfig_Buscreater/1 -> FrictionIDConfig/1
  Rate Transition120/1 -> Data Type Conversion103/1
  Const67/1 -> Rate Transition120/1
  Const1/1 -> Rate Transition1/1
  Rate Transition1/1 -> Data Type Conversion1/1
  Const2/1 -> Rate Transition2/1
  Rate Transition2/1 -> Data Type Conversion2/1
  Const3/1 -> Rate Transition3/1
  Rate Transition3/1 -> Data Type Conversion3/1
  Const65/1 -> Rate Transition117/1
  Const64/1 -> Rate Transition116/1
  Rate Transition116/1 -> Data Type Conversion99/1
  Rate Transition117/1 -> Data Type Conversion100/1
  Const69/1 -> Rate Transition122/1
  Rate Transition122/1 -> Data Type Conversion105/1
  TwoMassIDConfig_Buscreater/1 -> TwoMassIDConfig/1
  Const91/1 -> Rate Transition217/1
  Rate Transition217/1 -> Data Type Conversion134/1
  Data Type Conversion134/1 -> TwoMassIDConfig_Buscreater/1  "ScaleTorquePRBS"
  Rate Transition218/1 -> Data Type Conversion135/1
  n_ref measurement1/1 -> Rate Transition218/1
  Data Type Conversion135/1 -> TwoMassIDConfig_Buscreater/2  "n_ref_measurement"
  Rate Transition219/1 -> Data Type Conversion136/1
  Const93/1 -> Rate Transition220/1
  Const92/1 -> Rate Transition219/1
  Rate Transition220/1 -> Data Type Conversion137/1
  Data Type Conversion137/1 -> TwoMassIDConfig_Buscreater/3  "f_max"
  Data Type Conversion136/1 -> TwoMassIDConfig_Buscreater/4  "f_min"
  Rate Transition221/1 -> Data Type Conversion138/1
  Rate Transition222/1 -> Data Type Conversion139/1
  Const94/1 -> Rate Transition221/1
  Const95/1 -> Rate Transition222/1
  Data Type Conversion138/1 -> TwoMassIDConfig_Buscreater/5  "UseLbMq"
  Data Type Conversion139/1 -> TwoMassIDConfig_Buscreater/6  "d_TMS_start"
  FluxMapIDConfig_Buscreater/1 -> FluxMapIDConfig/1
  Rate Transition172/1 -> Data Type Conversion121/1
  Const80/1 -> Rate Transition171/1
  Const84/1 -> Rate Transition175/1
  Rate Transition175/1 -> Data Type Conversion124/1
  Rate Transition171/1 -> Data Type Conversion120/1
  Rate Transition174/1 -> Data Type Conversion123/1
  Const78/1 -> Rate Transition169/1
  Const82/1 -> Rate Transition173/1
  Const81/1 -> Rate Transition172/1
  Rate Transition169/1 -> Data Type Conversion118/1
  Rate Transition173/1 -> Data Type Conversion122/1
  Const83/1 -> Rate Transition174/1
  Data Type Conversion118/1 -> FluxMapIDConfig_Buscreater/1  "AMMsampleTime"
  Data Type Conversion120/1 -> FluxMapIDConfig_Buscreater/2  "IDstart"
  Rate Transition5/1 -> Data Type Conversion5/1
  Rate Transition6/1 -> Data Type Conversion6/1
  Const6/1 -> Rate Transition6/1
  Const4/1 -> Rate Transition4/1
  Const5/1 -> Rate Transition5/1
  Rate Transition4/1 -> Data Type Conversion4/1
  Data Type Conversion121/1 -> FluxMapIDConfig_Buscreater/3  "IDstepsize"
  Data Type Conversion122/1 -> FluxMapIDConfig_Buscreater/4  "IDstop"
  Data Type Conversion123/1 -> FluxMapIDConfig_Buscreater/5  "IQstart"
  Data Type Conversion124/1 -> FluxMapIDConfig_Buscreater/6  "IQstepsize"
  Data Type Conversion4/1 -> FluxMapIDConfig_Buscreater/7  "IQstop"
  Data Type Conversion5/1 -> FluxMapIDConfig_Buscreater/8  "R_s_ref"
  Data Type Conversion6/1 -> FluxMapIDConfig_Buscreater/9  "Temp_ref"
  ElectricalIDConfig_Buscreater/1 -> ElectricalIDConfig/1
  OnlineIDConfig_Buscreater/1 -> OnlineIDConfig/1
  Const37/1 -> Rate Transition52/1
  Rate Transition52/1 -> Data Type Conversion56/1
  Data Type Conversion56/1 -> OnlineIDConfig_Buscreater/2  "Temp_ref"
  Data Type Conversion77/1 -> OnlineIDConfig_Buscreater/4  "dev_curr"
  Data Type Conversion76/1 -> OnlineIDConfig_Buscreater/3  "dev_omega"
  Const44/1 -> Rate Transition73/1
  Const43/1 -> Rate Transition72/1
  Rate Transition72/1 -> Data Type Conversion76/1
  Const47/1 -> Rate Transition76/1
  Rate Transition73/1 -> Data Type Conversion77/1
  Rate Transition76/1 -> Data Type Conversion80/1
  Data Type Conversion80/1 -> OnlineIDConfig_Buscreater/5  "identRAmp"
  Data Type Conversion61/1 -> OnlineIDConfig_Buscreater/6  "AverageTransParams"
  Const28/1 -> Rate Transition79/1
  Rate Transition79/1 -> Data Type Conversion61/1
  Const56/1 -> Rate Transition94/1
  Data Type Conversion93/1 -> OnlineIDConfig_Buscreater/9  "allowPsiCalcOutside"
  Rate Transition94/1 -> Data Type Conversion91/1
  Data Type Conversion95/1 -> OnlineIDConfig_Buscreater/11  "max_n_ratio"
  Const58/1 -> Rate Transition96/1
  Const57/1 -> Rate Transition95/1
  Data Type Conversion91/1 -> OnlineIDConfig_Buscreater/7  "nom_factor"
  Rate Transition98/1 -> Data Type Conversion95/1
  Data Type Conversion92/1 -> OnlineIDConfig_Buscreater/8  "Rs_time"
  Rate Transition96/1 -> Data Type Conversion93/1
  Const59/1 -> Rate Transition97/1
  Rate Transition97/1 -> Data Type Conversion94/1
  Const60/1 -> Rate Transition98/1
  Data Type Conversion94/1 -> OnlineIDConfig_Buscreater/10  "min_n_ratio"
  Rate Transition95/1 -> Data Type Conversion92/1
  Rate Transition26/1 -> Data Type Conversion26/1
  Data Type Conversion26/1 -> OnlineIDConfig_Buscreater/1  "OnlineID_Reset"
  Const10/1 -> Rate Transition26/1
  Data Type Conversion11/1 -> FluxMapIDConfig_Buscreater/11  "identR"
  0 = off 1 = ident R_s online/1 -> Rate Transition11/1
  Rate Transition10/1 -> Data Type Conversion9/1
  Amplitude for SquareWave signal in d-current2/1 -> Rate Transition10/1
  Data Type Conversion9/1 -> FluxMapIDConfig_Buscreater/12  "identRAmp"
  Rate Transition11/1 -> Data Type Conversion11/1
  Data Type Conversion8/1 -> FluxMapIDConfig_Buscreater/10  "start_FM_ID"
  Rate Transition9/1 -> Data Type Conversion8/1
  Enable output/1 -> Rate Transition9/1
  Rate Transition23/1 -> Data Type Conversion23/1
  Const11/1 -> Rate Transition23/1
  Data Type Conversion23/1 -> OnlineIDConfig_Buscreater/12  "array_cleaned"
  Constant4/1 -> Rate Transition88/1
  Rate Transition88/1 -> Cast To Single/1
  Rate Transition24/1 -> Cast To Single1/1
  Constant3/1 -> Rate Transition24/1
  Rate Transition33/1 -> Cast To Single2/1
  Constant/1 -> Rate Transition33/1
  Rate Transition34/1 -> Cast To Single3/1
  Cast To Single3/1 -> AutoRefCurrentsConfig_Buscreator/1  "enableCRS"
  Activate ControlReference/1 -> Rate Transition34/1
  Rate Transition35/1 -> Cast To Single4/1
  Reset ControlReference/1 -> Rate Transition35/1
  Cast To Single4/1 -> AutoRefCurrentsConfig_Buscreator/2  "Reset"
  Cast To Single/1 -> AutoRefCurrentsConfig_Buscreator/3  "iq_points"
  Cast To Single1/1 -> AutoRefCurrentsConfig_Buscreator/4  "id_points"
  Cast To Single2/1 -> AutoRefCurrentsConfig_Buscreator/5  "max_current"
  AutoRefCurrentsConfig_Buscreator/1 -> AutoRefCurrentsconfig/1
  Rate Transition18/1 -> Data Type Conversion17/1
  Data Type Conversion17/1 -> ElectricalIDConfig_Buscreater/1  "goertzlFreq"
  goertzlFreq in Hz/1 -> Rate Transition18/1
  Rate Transition8/1 -> Data Type Conversion7/1
  Const20/1 -> Rate Transition48/1
  Data Type Conversion14/1 -> ElectricalIDConfig_Buscreater/3  "n_ref_measurement"
  manual input of a DutyCycle/1 -> Rate Transition8/1
  "0 = Lq=Ld 1 = identify Lq "/1 -> Rate Transition7/1
  Const62/1 -> Rate Transition100/1
  n_ref measurement/1 -> Rate Transition12/1
  Data Type Conversion7/1 -> ElectricalIDConfig_Buscreater/2  "dutyCyc"
  Data Type Conversion97/1 -> ElectricalIDConfig_Buscreater/6  "min_n_ratio"
  Rate Transition7/1 -> Data Type Conversion10/1
  Rate Transition48/1 -> Data Type Conversion52/1
  Rate Transition12/1 -> Data Type Conversion14/1
  Data Type Conversion52/1 -> ElectricalIDConfig_Buscreater/5  "goertzlTorque"
  Data Type Conversion10/1 -> ElectricalIDConfig_Buscreater/4  "identLq"
  Rate Transition100/1 -> Data Type Conversion97/1
  Rate Transition25/1 -> Data Type Conversion40/1
  Rate Transition62/1 -> Data Type Conversion58/1
  Const25/1 -> Rate Transition38/1
  Rate Transition51/1 -> Data Type Conversion46/1
  Data Type Conversion24/1 -> GlobalConfig_Buscreator1/3  "Reset"
  Data Type Conversion45/1 -> GlobalConfig_Buscreator1/20  "n_ref"
  ISR sample time 0.2/1 -> Rate Transition51/1
  Bus Creator2/1 -> GlobalConfig_Buscreator1/19  "i_dq_ref"
  Rate Transition50/1 -> Data Type Conversion45/1
  n_ref1/1 -> Rate Transition50/1
  Rate Transition55/1 -> Data Type Conversion49/1
  Rate Transition61/1 -> Data Type Conversion57/1
  Const12/1 -> Rate Transition41/1
  Rate Transition59/1 -> Data Type Conversion51/1
  3/1 -> Rate Transition59/1
  Rate Transition38/1 -> Data Type Conversion39/1
  Rate Transition46/1 -> Data Type Conversion37/1
  Const24/1 -> Rate Transition37/1
  Data Type Conversion38/1 -> Bus Creator1/3  "Lq_Henry"
  Data Type Conversion34/1 -> GlobalConfig_Buscreator1/8  "Ki_iq"
  Const14/1 -> Rate Transition62/1
  Rate Transition53/1 -> Data Type Conversion47/1
  Rate Transition41/1 -> Data Type Conversion42/1
  Bus Creator1/1 -> GlobalConfig_Buscreator1/1  "PMSM_config"
  Data Type Conversion42/1 -> Bus Creator1/4  "Psi_PM_Vs"
  Data Type Conversion41/1 -> GlobalConfig_Buscreator1/13  "FluxMapID"
  Rate Transition56/1 -> Data Type Conversion54/1
  Const13/1 -> Rate Transition61/1
  Data Type Conversion40/1 -> GlobalConfig_Buscreator1/12  "TwoMassID"
  Constant1/1 -> Rate Transition47/1
  Rate Transition47/1 -> Data Type Conversion43/1
  Data Type Conversion37/1 -> GlobalConfig_Buscreator1/9  "Ki_n"
  Data Type Conversion53/1 -> Bus Creator1/7  "I_max_Ampere"
  doTwoMassID1/1 -> Rate Transition25/1
  Data Type Conversion35/1 -> GlobalConfig_Buscreator1/7  "Ki_id"
  Data Type Conversion54/1 -> GlobalConfig_Buscreator1/10  "ElectricalID"
  Rate Transition45/1 -> Data Type Conversion36/1
  doFrictionID1/1 -> Rate Transition57/1
  Rate Transition36/1 -> Data Type Conversion41/1
  doElectricalID1/1 -> Rate Transition56/1
  Data Type Conversion55/1 -> GlobalConfig_Buscreator1/11  "FrictionID"
  Rate Transition43/1 -> Data Type Conversion34/1
  Rate Transition57/1 -> Data Type Conversion55/1
  Rate Transition39/1 -> Data Type Conversion24/1
  Const18/1 -> Rate Transition42/1
  Data Type Conversion47/1 -> GlobalConfig_Buscreator1/14  "OnlineID"
  Const21/1 -> Rate Transition44/1
  i_q1/1 -> Bus Creator2/2  "q"
  enableParameterID1/1 -> Rate Transition54/1
  Rate Transition44/1 -> Data Type Conversion35/1
  Const19/1 -> Rate Transition43/1
  Data Type Conversion49/1 -> Bus Creator1/2  "Ld_Henry"
  Number of pole pairs1/1 -> Rate Transition58/1
  Data Type Conversion50/1 -> Bus Creator1/5  "polePairs"
  Data Type Conversion46/1 -> GlobalConfig_Buscreator1/16  "sampleTimeISR"
  Rate Transition54/1 -> Data Type Conversion48/1
  Rate Transition58/1 -> Data Type Conversion50/1
  Data Type Conversion51/1 -> Bus Creator1/6  "J_kg_m_squared"
  Data Type Conversion58/1 -> GlobalConfig_Buscreator1/18  "ratSpeed"
  Data Type Conversion57/1 -> GlobalConfig_Buscreator1/17  "ratCurrent"
  Rate Transition42/1 -> Data Type Conversion33/1
  Data Type Conversion43/1 -> GlobalConfig_Buscreator1/15  "ACCEPT"
  i_d1/1 -> Bus Creator2/1  "d"
  Data Type Conversion48/1 -> GlobalConfig_Buscreator1/2  "enableParameterID"
  Data Type Conversion39/1 -> Bus Creator1/1  "R_ph_Ohm"
  GlobalConfig_Buscreator1/1 -> GlobalConfig/1
  i_zero1/1 -> Bus Creator2/3  "zero"
  Rate Transition37/1 -> Data Type Conversion38/1
  1 = reset1/1 -> Rate Transition39/1
  Data Type Conversion25/1 -> GlobalConfig_Buscreator1/4  "Kp_id"
  doFluxMapID1/1 -> Rate Transition36/1
  Rate Transition40/1 -> Data Type Conversion25/1
  Const16/1 -> Rate Transition55/1
  Data Type Conversion33/1 -> GlobalConfig_Buscreator1/5  "Kp_iq"
  Data Type Conversion36/1 -> GlobalConfig_Buscreator1/6  "Kp_n"
  Const22/1 -> Rate Transition45/1
  enableOnlineID1/1 -> Rate Transition53/1
  Const23/1 -> Rate Transition46/1
  Rate Transition60/1 -> Data Type Conversion53/1
  Const17/1 -> Rate Transition40/1
  2/1 -> Rate Transition60/1
  n_ref2/1 -> Rate Transition13/1
  Rate Transition13/1 -> Data Type Conversion12/1
  Data Type Conversion12/1 -> GlobalConfig_Buscreator1/21  "voltage_measurement_C"
  Data Type Conversion13/1 -> GlobalConfig_Buscreator1/22  "voltage_measurement_Rp"
  Rate Transition14/1 -> Data Type Conversion13/1
  n_ref3/1 -> Rate Transition14/1
  n_ref4/1 -> Rate Transition15/1
  Rate Transition15/1 -> Data Type Conversion15/1
  Data Type Conversion15/1 -> GlobalConfig_Buscreator1/23  "voltage_measurement_Rs"
